simulink model "Simulation"  (R2020b)
settings: Solver=VariableStepAuto  StartTime=0.0  StopTime=10.0  RelTol=1e-3
libraries: simulink x1
settings Model: Creator=elbit  LastModifiedBy=alons

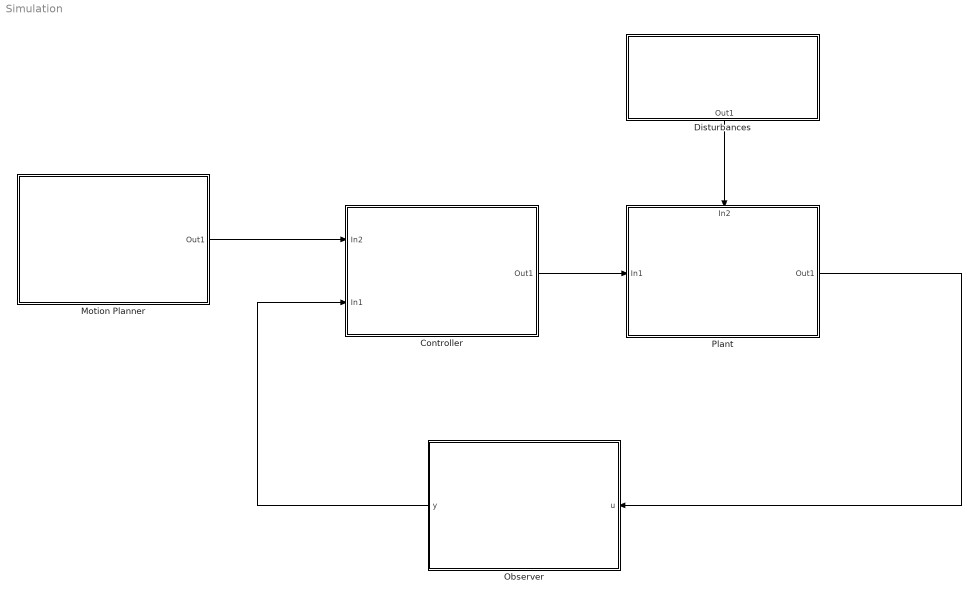
== system Simulation ==
  Controller : Subsystem
  Disturbances : Subsystem
      settings: PortSchema="{\"entries\":[{\"content\":{\"sides\":[{\"content\":{\"connectorIds\":[]},\"type\":\"ConnectorPlacement.EquallySpacedRectSide\",\"uuid\":\"9b33d3af-0c8d-4b96-90d4-8e7d863823ff\"},{\"content\":{\"connectorIds\":[],\"side\":\"RIGHT\"},\"type\":\"ConnectorPlacement.EquallySpacedRectSide\",\"uuid\":\"cdb3a2a1-2d18-474f-9929-620728e89e35\"},{\"content\":{\"connectorIds\":[],\"side\":\"TOP\"},\"type\":\"ConnectorPlacement.EquallySpacedRectSide\",\"uuid\":\"b20622dc-cbfb-482f-9e47-a1277a697cb0\"},{\"content\":{\"connectorIds\":[\"Out1\"],\"side\":\"BOTTOM\"},\"type\":\"ConnectorPlacement.EquallySpacedRectSide\",\"uuid\":\"7af72e98-18a2-44d9-8ff7-e17ff6a4dcec\"},{\"content\":{\"connectorIds\":[],\"side\":\"HIDDEN\"},\"type\":\"ConnectorPlacement.EquallySpacedRectSide\",\"uuid\":\"dc9e3ef7-abc5-47dc-a3d7-4e2143ad8265\"}]},\"type\":\"ConnectorPlacement.EquallySpacedConnector\",\"uuid\":\"af3e8111-2b67-43ec-9e73-baa4ec12e35e\"}],\"packageUris\":[\"http://schema.mathworks.com/mf0/Connector/R2020b\"],\"version\":\"1.0\"}"
  Motion Planner : Subsystem
  Observer : Subsystem
  Plant : Subsystem
      settings: PortSchema="{\"entries\":[{\"content\":{\"sides\":[{\"content\":{\"connectorIds\":[\"In1\"]},\"type\":\"ConnectorPlacement.EquallySpacedRectSide\",\"uuid\":\"4b842b0f-12d4-4db1-a761-d4dd788a733f\"},{\"content\":{\"connectorIds\":[\"Out1\"],\"side\":\"RIGHT\"},\"type\":\"ConnectorPlacement.EquallySpacedRectSide\",\"uuid\":\"23ba60fa-688b-44ce-8b48-688e6347ad39\"},{\"content\":{\"connectorIds\":[\"In2\"],\"side\":\"TOP\"},\"type\":\"ConnectorPlacement.EquallySpacedRectSide\",\"uuid\":\"897a919d-7c9a-40f6-aa86-e062506864f0\"},{\"content\":{\"connectorIds\":[],\"side\":\"HIDDEN\"},\"type\":\"ConnectorPlacement.EquallySpacedRectSide\",\"uuid\":\"43c05ff6-1092-494d-92a9-cce0f4983a94\"}]},\"type\":\"ConnectorPlacement.EquallySpacedConnector\",\"uuid\":\"59635b9b-a907-4eea-bec0-53190ded3b3c\"}],\"packageUris\":[\"http://schema.mathworks.com/mf0/Connector/R2020b\"],\"version\":\"1.0\"}"
  wires:
  Controller/1(Out1) -> Plant/1(In1)
  Motion Planner/1(Out1) -> Controller/1(In2)
  Plant/1(Out1) -> Observer/1(u)
  Observer/1(y) -> Controller/2(In1)
  Disturbances/1(Out1) -> Plant/2(In2)

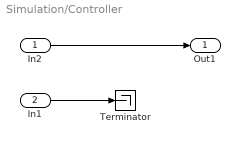
== system Simulation/Controller ==
  In2 : Inport
  In1 : Inport  Port=2
  Terminator : Terminator
  Out1 : Outport
  wires:
  In2/1 -> Out1/1
  In1/1 -> Terminator/1

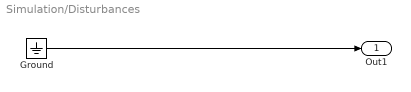
== system Simulation/Disturbances ==
  Ground : Ground
  Out1 : Outport
  wires:
  Ground/1 -> Out1/1

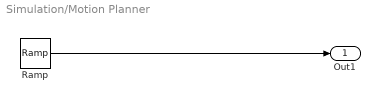
== system Simulation/Motion Planner ==
  Ramp : simulink/Sources/Ramp  slope=1  start=0  InitialOutput=0
  Out1 : Outport
  wires:
  Ramp/1 -> Out1/1

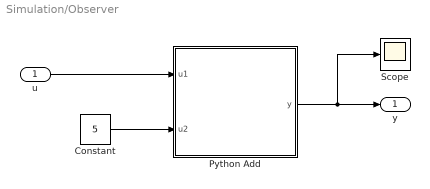
== system Simulation/Observer ==
  u : Inport
  Constant : Constant  Value=5
  Python Add : MATLAB Function  TreatAsAtomicUnit=on
  Scope : Scope
  y : Outport
  wires:
  u/1 -> Python Add/1(u1)
  Python Add/1(y) -> Scope/1, y/1
  Constant/1 -> Python Add/2(u2)

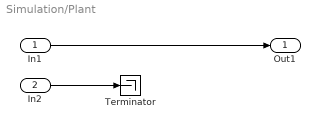
== system Simulation/Plant ==
  In1 : Inport
  In2 : Inport  Port=2
  Terminator : Terminator
  Out1 : Outport
  wires:
  In1/1 -> Out1/1
  In2/1 -> Terminator/1

== matlab function Simulation/Observer/Python Add ==
  data: u1 input; y output; u2 input
function y = RunPython(u1,u2)
y = 0; % Has to be preassigned, otherwise Simulink throws an error
coder.extrinsic('py.Test.pyhon_add')  % Python functions have to be run extrinsically, meaning no C code generated
y = py.Test.pyhon_add(u1,u2);
